simulink model "sim_model"  (R2023b)
settings: Solver=VariableStepAuto  StartTime=0.0  StopTime=10.0  MaxStep=5  RelTol=1e-3
undefined symbols (not defined in the file): delta_Twew_SP, ki, kp, T_wew0, t_wew_SP, T_wew_SP_0
libraries: cstblocks x1
settings Model: Creator=tomasz  LastModifiedBy=tomasz

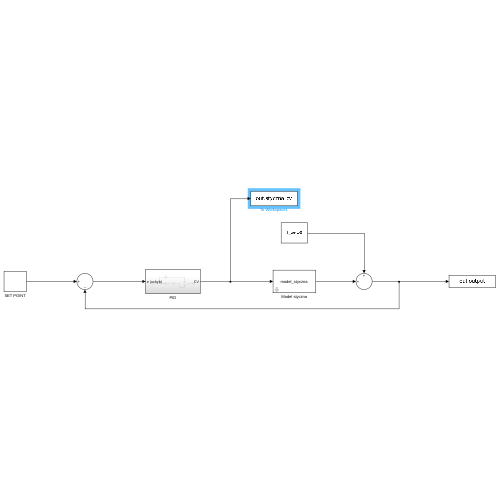
[thumbnail: Simulink's stored preview of the top-level diagram]
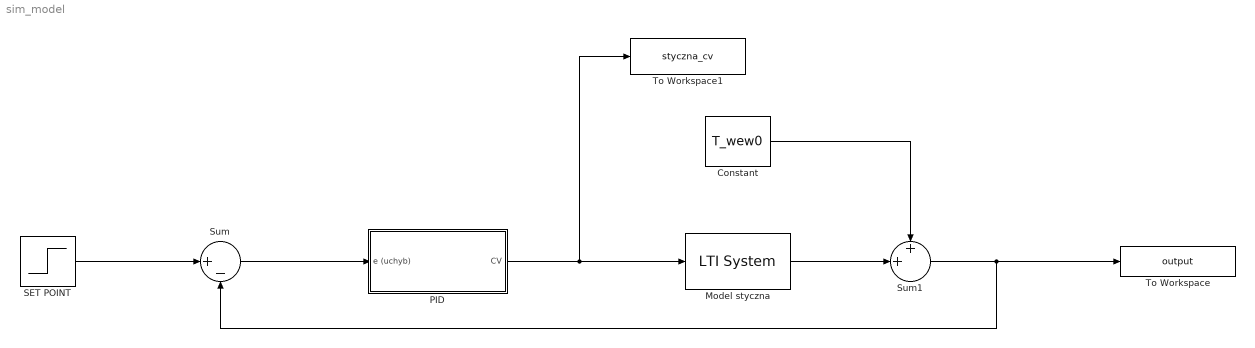
== system sim_model ==
  Constant : Constant  Value=T_wew0
  Model styczna : cstblocks/LTI System  sys=model_styczna  IC=[]  PadeOrder=0
  PID : Subsystem
  SET POINT : Step  Time=t_wew_SP  Before=T_wew_SP_0  After=T_wew_SP_0 + delta_Twew_SP  SampleTime=0
  Sum : Sum  Inputs=|+-
  Sum1 : Sum  Inputs=++|
  To Workspace : ToWorkspace  VariableName=output  SampleTime=-1
  To Workspace1 : ToWorkspace  VariableName=styczna_cv  SampleTime=-1
  wires:
  PID/1(CV) -> To Workspace1/1, Model styczna/1
  Sum/1 -> PID/1(e (uchyb))
  Model styczna/1 -> Sum1/2
  Sum1/1 -> Sum/2, To Workspace/1
  SET POINT/1 -> Sum/1
  Constant/1 -> Sum1/1

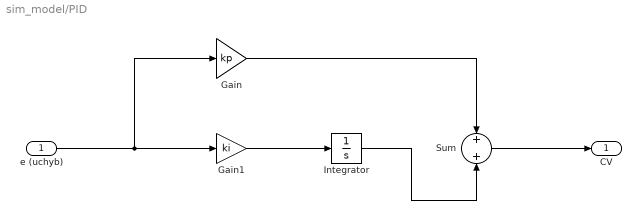
== system sim_model/PID ==
  e (uchyb) : Inport
  Gain : Gain  Gain=kp
  Gain1 : Gain  Gain=ki
  Integrator : Integrator
  Sum : Sum
  CV : Outport
  wires:
  Integrator/1 -> Sum/2
  Gain1/1 -> Integrator/1
  Gain/1 -> Sum/1
  e (uchyb)/1 -> Gain1/1, Gain/1
  Sum/1 -> CV/1
